simulink model "MATLAB_TEST"  (R2019b)
settings: Solver=FixedStepDiscrete  StartTime=0  StopTime=50  FixedStep=0.0025  RelTol=1e-3
undefined symbols (not defined in the file): BCM_COM_PROC_P20, BCM_COM_PROC_P20_SFW_R2018b, BCM_COM_PROC_P2_5, BCM_COM_PROC_P2_5_SFW_R2018b, BCM_COM_PROC_P5, BCM_COM_PROC_P5_SFW_R2018b, BCMA_ACCU_PT_Conf_Flt, BCMA_ACCU_PT_Unconf_Flt, BCMA_Antiskid_Off_Sanction, BCMA_Avionics_Conf_Flt, BCMA_BCM_CCDL_Conf_Flt, BCMA_BCM_CCDL_Unconf_Flt, BCMA_BCM_DBCU_INHIBITION_Conf_Flt, BCMA_BCM_DBCU_INHIBITION_Unconf_Flt, BCMA_BCP_ALT_Disp_Sw_Conf_Flt, BCMA_BCP_ALT_Disp_Sw_Unconf_Flt, BCMA_BCP_ALT_SW_ON_CMD_Conf_Flt, BCMA_BCP_ALT_SW_ON_CMD_Unconf_Flt, BCMA_BCP_PARK_OFF_SW_CMD_Conf_Flt, BCMA_BCP_PARK_OFF_SW_CMD_Unconf_Flt, BCMA_CF_BSELV_JCL, BCMA_CF_BSELV_JOP, BCMA_CF_BSELV_OC, BCMA_CF_BSELV_SC, BCMA_CF_LH_SV_JCL, BCMA_CF_LH_SV_JOP, BCMA_CF_LH_SV_OC, BCMA_CF_LH_SV_SC, BCMA_CF_PARK_BRK, BCMA_CF_RESIDUAL_PRESS, BCMA_CF_RH_SV_JCL, BCMA_CF_RH_SV_JOP, BCMA_CF_RH_SV_OC, BCMA_CF_RH_SV_SC, BCMA_CF_SELV_JCL, BCMA_CF_SELV_JOP, BCMA_CF_SELV_OC, BCMA_CF_SELV_SC, BCMA_CF_SV_DRIFT, BCMA_DBCU_ALT_MODE_Conf_Flt, BCMA_DBCU_ALT_MODE_Unconf_Flt, BCMA_DBCU_BRK_ORDER_FAIL_Conf_Flt, BCMA_DBCU_BRK_ORDER_FAIL_Unconf_Flt, BCMA_DBCU_Conf_Flt, BCMA_DBCU_DISPATCH_SW_ON_Conf_Flt, BCMA_DBCU_DISPATCH_SW_ON_Unconf_Flt, BCMA_DBCU_FAILED_Conf_Flt, BCMA_DBCU_FAILED_Unconf_Flt, BCMA_DFCS1_Capsule_Validity, BCMA_DFCS1_Label202_Corrupted, BCMA_DFCS1_Label202_Not_Refreshed, BCMA_DFCS1_Label204_Corrupted, BCMA_DFCS1_Label204_Not_Refreshed, BCMA_DFCS1_Label205_Corrupted, BCMA_DFCS1_Label205_Not_Refreshed, BCMA_DFCS1_Label206_Corrupted, BCMA_DFCS1_Label206_Not_Refreshed, BCMA_DFCS1_Label207_Corrupted, BCMA_DFCS1_Label207_Not_Refreshed, BCMA_DFCS3_Capsule_Validity ... (+762)
libraries: simulink x73, lib_MBD_Control x5
(part 1 of 16)
settings Model: Creator=C057006  LastModifiedBy=FX622208
settings DataIOCC: ReturnWorkspaceOutputs=off
settings OptimizationCC: DefaultParameterBehavior=Inlined
settings DebuggingCC: ParameterPrecisionLossMsg=none  BusObjectLabelMismatch=error  ArithmeticOperatorsInVariantConditions=warning
settings HardwareCC: TargetBitPerLong=64  TargetIntDivRoundTo=Zero  TargetEndianess=LittleEndian  TargetPreprocMaxBitsSint=64  TargetPreprocMaxBitsUint=64  TargetHWDeviceType=Custom Processor->Custom Processor  ProdEqTarget=off
settings SFSimCC: SimUseLocalCustomCode=off  CustomCodeUndefinedFunction=UseInterfaceOnly
settings RTWCC: Description=rtc_Linux_x86_64  SystemTargetFile=rtc_linux_x86_64.tlc  TemplateMakefile=rtc_linux.tmf  RetainRTWFile=on  RTWUseLocalCustomCode=off
settings CodeAppCC: MaxIdLength=127  StateflowObjectComments=on
settings GRTTargetCC: UseToolchainInfoCompliant=off
settings SimscapeCC: SimscapeNormalizeSystem=off

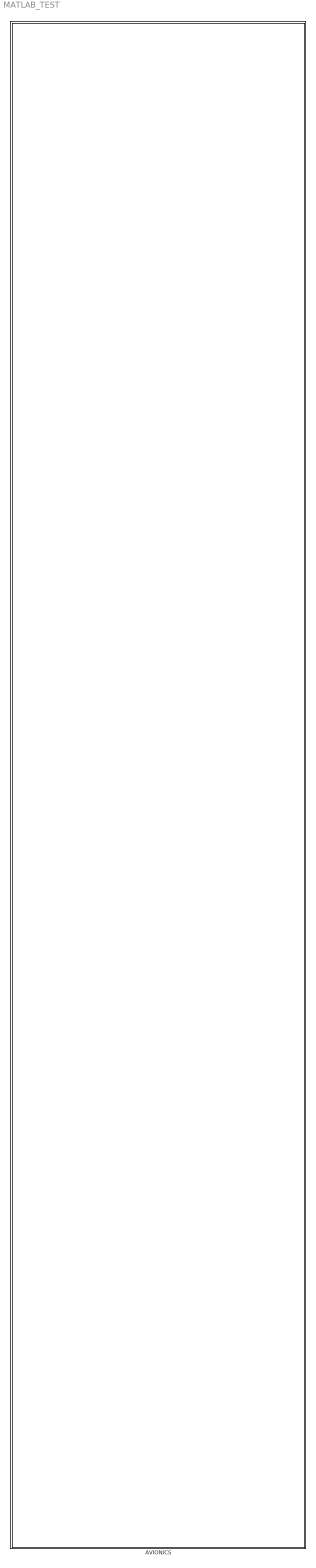
== system MATLAB_TEST ==
  AVIONICS : Subsystem

== system MATLAB_TEST/AVIONICS ==
  Brake_Control_Module_Side_A : Subsystem

== system MATLAB_TEST/AVIONICS/Brake_Control_Module_Side_A ==
  BCSA Controller CP : Subsystem
  Unit Delay : UnitDelay  SampleTime=-1  HasFrameUpgradeWarning=on
  Unit Delay1 : UnitDelay  SampleTime=-1  HasFrameUpgradeWarning=on
  Unit Delay2 : UnitDelay  SampleTime=-1  HasFrameUpgradeWarning=on
  wires:
  [BCP_ALT_SW_ON_CMD_BCM_A_GND] -> BCSA Controller CP/1(BCP_ALT_SW_ON_CMD_BCM_A_GND)
  [BCP_PARK_OFF_SW_CMD_BCM_A_GND] -> BCSA Controller CP/2(BCP_PARK_OFF_SW_CMD_BCM_A_GND)
  [BUS_A429_DFCS1_BCMA] -> BCSA Controller CP/3(BUS_A429_DFCS1_BCMA)
  [BUS_A429_DFCS3_BCMA] -> BCSA Controller CP/4(BUS_A429_DFCS3_BCMA)
  [BUS_A429_GenIO_1A_GPHS] -> BCSA Controller CP/5(BUS_A429_GenIO_1A_GPHS)
  [LGCH_LG_LEVER_UP_1] -> BCSA Controller CP/10(LGCH_LG_LEVER_UP_1)
  [LH_ESC_WOnWdiscrete] -> BCSA Controller CP/11(LH_ESC_WOnWdiscrete)
  [LMLG_DOWN_LOCKED_BCM_1] -> BCSA Controller CP/12(LMLG_DOWN_LOCKED_BCM_1)
  [MP_MAINT_MODE_CMD_BCM_A_28V] -> BCSA Controller CP/13(MP_MAINT_MODE_CMD_BCM_A_28V)
  [MP_MAINT_MODE_CMD_BCM_A_GND] -> BCSA Controller CP/14(MP_MAINT_MODE_CMD_BCM_A_GND)
  [RMLG_DOWN_LOCKED_BCM_1] -> BCSA Controller CP/15(RMLG_DOWN_LOCKED_BCM_1)
  [ACCU_PT_PRESSURE] -> BCSA Controller CP/16(ACCU_PT_PRESSURE)
  [BCMB_DBCU_INHIBITION] -> BCSA Controller CP/17(BCMB_DBCU_INHIBITION)
  [DBCU_ALTERNATE_MODE_1] -> BCSA Controller CP/18(DBCU_ALTERNATE_MODE_1)
  [DBCU_BRK_ORDER_FAIL_BCMA] -> BCSA Controller CP/19(DBCU_BRK_ORDER_FAIL_BCMA)
  [DBCU_FAILED_BCMA] -> BCSA Controller CP/20(DBCU_FAILED_BCMA)
  [LH_DBCU_BRK_CMD_FEEDBACK] -> BCSA Controller CP/21(LH_DBCU_BRK_CMD_FEEDBACK)
  [LH_HASV_PT_PRESSURE] -> BCSA Controller CP/22(LH_HASV_PT_PRESSURE)
  [LH_IN_WHEEL_SPEED_COIL1] -> BCSA Controller CP/23(LH_IN_WHEEL_SPEED_COIL1)
  [LH_OUT_BTS_TEMP] -> BCSA Controller CP/24(LH_OUT_BTS_TEMP)
  [LH_OUT_WHEEL_SPEED_COIL1] -> BCSA Controller CP/25(LH_OUT_WHEEL_SPEED_COIL1)
  [PBSELV_ON_POS] -> BCSA Controller CP/26(PBSELV_ON_POS)
  [RH_DBCU_BRK_CMD_FEEDBACK] -> BCSA Controller CP/27(RH_DBCU_BRK_CMD_FEEDBACK)
  [RH_HASV_PT_PRESSURE] -> BCSA Controller CP/28(RH_HASV_PT_PRESSURE)
  [RH_IN_WHEEL_SPEED_COIL1] -> BCSA Controller CP/29(RH_IN_WHEEL_SPEED_COIL1)
  [RH_OUT_BTS_TEMP] -> BCSA Controller CP/30(RH_OUT_BTS_TEMP)
  [RH_OUT_WHEEL_SPEED_COIL1] -> BCSA Controller CP/31(RH_OUT_WHEEL_SPEED_COIL1)
  BCSA Controller CP/1(BUS_A429_BCMA_DFCS13) -> [BUS_A429_BCMA_DFCS13]
  BCSA Controller CP/5(BCMA_DBCU_INHIBITION) -> [BCMA_DBCU_INHIBITION_CP]
  BCSA Controller CP/6(HASELV_CMD) -> [HASELV_CMD_CP]
  BCSA Controller CP/7(LH_HASV_CURRENT) -> [LH_HASV_CURRENT_CP]
  BCSA Controller CP/8(RH_HASV_CURRENT) -> [RH_HASV_CURRENT_CP]
  BCSA Controller CP/2(BUS_A429_BCMA_GenIO_2) -> [BUS_A429_BCMA_GenIO_2]
  BCSA Controller CP/3(BUS_ETH_BCMA_MMS) -> [BUS_ETH_BCMA_MMS]
  [BUS_ETH_MMS_BCMA] -> BCSA Controller CP/8(BUS_ETH_MMS_BCMA)
  [BUS_CAN_BCM_CCDL_RX] -> BCSA Controller CP/9(BUS_CAN_BCM_CCDL_RX)
  BCSA Controller CP/4(BUS_CAN_BCM_CCDL) -> [BUS_CAN_BCM_CCDL]
  [FTI_BCMA_switch_1] -> BCSA Controller CP/32(FTI_BCMA_switch_1)
  [FTI_BCMA_switch_2] -> BCSA Controller CP/33(FTI_BCMA_switch_2)
  [FTI_BCMA_switch_3] -> BCSA Controller CP/34(FTI_BCMA_switch_3)
  [FTI_BCMA_switch_4] -> BCSA Controller CP/35(FTI_BCMA_switch_4)
  [FTI_BCMA_switch_5] -> BCSA Controller CP/36(FTI_BCMA_switch_5)
  [PIN_PROG_BCMA_1] -> BCSA Controller CP/37(PIN_PROG_BCMA_1)
  [PIN_PROG_BCMA_2] -> BCSA Controller CP/38(PIN_PROG_BCMA_2)
  [PIN_PROG_BCMA_3] -> BCSA Controller CP/39(PIN_PROG_BCMA_3)
  [BUS_A429_LH_WRDC_BCM] -> BCSA Controller CP/6(BUS_A429_LH_WRDC_BCM)
  [BUS_A429_RH_WRDC_BCM] -> BCSA Controller CP/7(BUS_A429_RH_WRDC_BCM)
  [MON_CAN_COM] -> BCSA Controller CP/40(MON_CAN_COM)
  [Control_Path_Start_Up] -> BCSA Controller CP/41(Control_Path_Start_Up)
  Unit Delay/1 -> BCSA Controller CP/42(LH_HASV_CURRENT_COIL1_Readback)
  [LH_HASV_CURRENT_COIL1_Readback] -> Unit Delay/1
  [RH_HASV_CURRENT_COIL1_Readback] -> Unit Delay1/1
  Unit Delay1/1 -> BCSA Controller CP/43(RH_HASV_CURRENT_COIL1_Readback)
  [HASELV_CMD_Readback] -> Unit Delay2/1
  Unit Delay2/1 -> BCSA Controller CP/44(HASELV_CMD_Readback)
